simulink model "inverted_pendulum_kalman"  (R2016b)
settings: Solver=VariableStepAuto  StartTime=0.0  StopTime=10  RelTol=1e-3
settings Model: Creator=Quy  LastModifiedBy=Anass

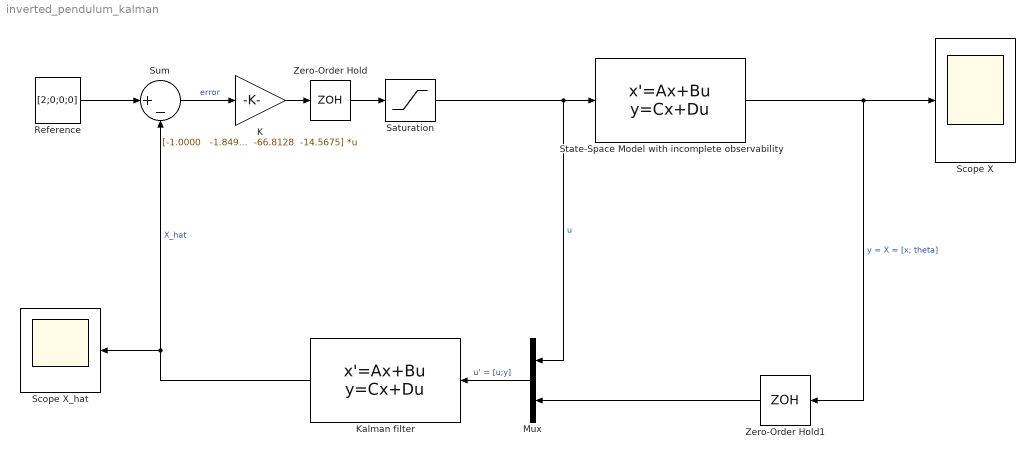
== system inverted_pendulum_kalman ==
  K : Gain  Gain="[-1.0000   -1.8497  -66.8128  -14.5675]"  Multiplication=Matrix(K*u) (u vector)
  Kalman filter : StateSpace  A=|  B=|  C=eye(4)  D=zeros(4,3)  X0=[1; 0; 0; 0]
      A=|
      | [   -3.0367    1.0000    0.0678         0;
      |    -4.6131  -10.4100    0.9845         0;
      |     0.0678         0  -11.5434    1.0000;
      |     0.0035    4.3111  -29.8872   -0.6249]
      B=|
      | [         0    3.0367   -0.0678;
      |    51.2860    4.6131   -0.9845;
      |          0   -0.0678   11.5434;
      |   -21.0230   -0.0035   66.6272]
  Mux : Mux  Inputs=2
  Reference : Constant  Value=[2;0;0;0]
  Saturation : Saturate  UpperLimit=0.9  LowerLimit=-0.8
  Scope X : Scope
  Scope X_hat : Scope
  State-Space Model with incomplete observability : StateSpace  A=|  B=|  C=[1 0 0 0;0 0 1 0]  D=[0; 0]  X0=[1; 0; 0.1; 0]
      A=|
      | [0    1.0000         0         0;
      |          0  -10.4100         0         0;
      |          0         0         0    1.0000;
      |          0    4.3111   36.7400   -0.6249]
      B=|
      | [0;
      |    51.2860;
      |          0;
      |   -21.0230]
  Sum : Sum  Inputs=|+-
  Zero-Order Hold : ZeroOrderHold  SampleTime=0.01
  Zero-Order Hold1 : ZeroOrderHold  SampleTime=0.01
  wires:
  State-Space Model with incomplete observability/1 -> Zero-Order Hold1/1, Scope X/1  "y = X = [x; theta]"
  Sum/1 -> K/1  "error"
  Reference/1 -> Sum/1
  K/1 -> Zero-Order Hold/1
  Zero-Order Hold/1 -> Saturation/1
  Kalman filter/1 -> Sum/2, Scope X_hat/1  "X_hat"
  Zero-Order Hold1/1 -> Mux/2
  Mux/1 -> Kalman filter/1  "u' = [u;y]"
  Saturation/1 -> Mux/1, State-Space Model with incomplete observability/1  "u"
